simulink model "Simulation_Example"  (R2017b)
settings: Solver=VariableStepAuto  StartTime=0.0  StopTime=60  RelTol=1e-3
libraries: SY202_NCS_Library x9
settings Model: Creator=rodrigue  LastModifiedBy=rodrigue

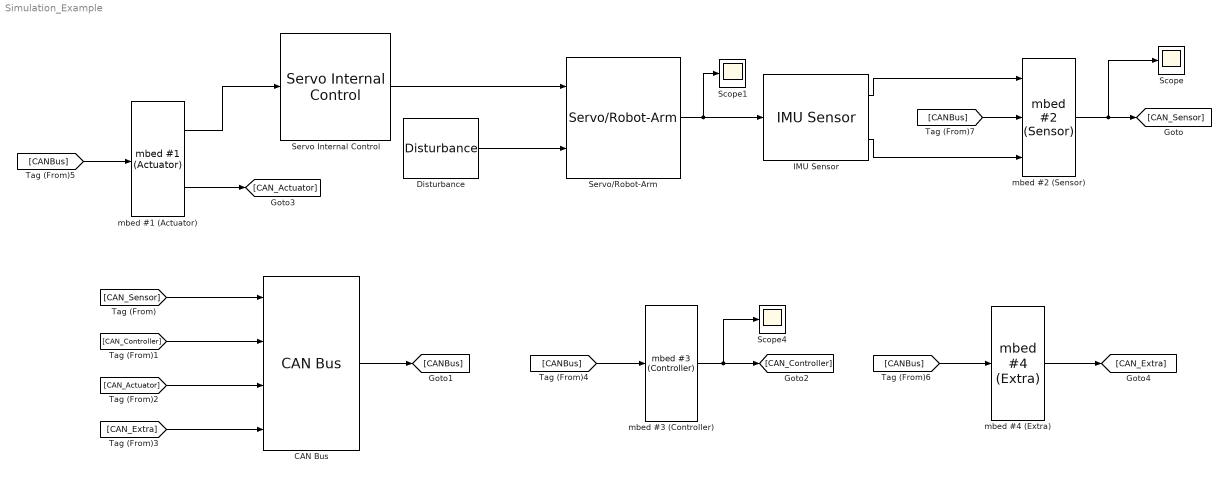
== system Simulation_Example ==
  CAN Bus : SY202_NCS_Library/CAN Bus
  Disturbance : SY202_NCS_Library/Disturbance  DisturbanceTime=0  DisturbanceValue=0
  IMU Sensor : SY202_NCS_Library/IMU Sensor  MeanSensorError=0  MeanSensorVar=0.002
  Scope : Scope
  Scope1 : Scope
  Scope4 : Scope
  Servo Internal Control : SY202_NCS_Library/Servo Internal Control  MaxPW=2100  MinPW=900  MaxServo=pi/3  MinServo=-pi/3
  Servo/Robot-Arm : SY202_NCS_Library/Servo//Robot-Arm  x0=-.5  MaxPW=2100  MinPW=900  MaxServo=pi/3  MinServo=-pi/3
  mbed #1 (Actuator) : SY202_NCS_Library/mbed #1 (Actuator)  MinPW=900  MaxPW=2100
  mbed #2 (Sensor) : SY202_NCS_Library/mbed #2 (Sensor)
  mbed #3 (Controller) : SY202_NCS_Library/mbed #3 (Controller)  DesValue=0  Kp=100  Ki=250  Offset=1400
  mbed #4 (Extra) : SY202_NCS_Library/mbed #4 (Extra)  AttackRate=0  AttackMode=Stealth Attack  AttackMag=0.2  AttackTime=20
  wires:
  [CAN_Sensor] -> CAN Bus/1
  mbed #2 (Sensor)/1 -> Scope/1, [CAN_Sensor]
  [CAN_Controller] -> CAN Bus/2
  [CAN_Actuator] -> CAN Bus/3
  [CAN_Extra] -> CAN Bus/4
  CAN Bus/1 -> [CANBus]
  mbed #3 (Controller)/1 -> Scope4/1, [CAN_Controller]
  mbed #1 (Actuator)/2 -> [CAN_Actuator]
  mbed #4 (Extra)/1 -> [CAN_Extra]
  [CANBus] -> mbed #3 (Controller)/1
  [CANBus] -> mbed #1 (Actuator)/1
  [CANBus] -> mbed #4 (Extra)/1
  [CANBus] -> mbed #2 (Sensor)/2
  mbed #1 (Actuator)/1 -> Servo Internal Control/1
  Servo Internal Control/1 -> Servo/Robot-Arm/1
  Disturbance/1 -> Servo/Robot-Arm/2
  Servo/Robot-Arm/1 -> Scope1/1, IMU Sensor/1
  IMU Sensor/1 -> mbed #2 (Sensor)/1
  IMU Sensor/2 -> mbed #2 (Sensor)/3
